simulink model "PhaseII_opalrt_NoProtection"  (Simulink 8.8)
settings: Solver=ode3  StartTime=0.0  StopTime=inf  FixedStep=Ts  RelTol=1e-5  EnableMultiTasking=on
PostLoadFcn:
  | %BESS ctrl
  | Kpf=0.005*3*12;
  | Kif=5*6;
  | 
  | Kpf1=0.005*3*12;
  | Kif1=5*6;
  | Kp_v=0.016*15*35;
  | Ki_v=12*25;
  | 
  | Kp_v1=0.016*15*35;
  | Ki_v1=12*25;
  | 
  | Vabc_B=12.47e3;
  | Vdc_ref=Vabc_B*2;
  | Kpwm=sqrt(2)*Vabc_B/Vdc_ref;
  | ZB=Vabc_B^2/1e6;
  | R=0.005*ZB;
  | Ibasefull=673/2*sqrt(2);
  | 
  | 
  | Ts_Control=1e-4;
  | ts=0.05;
  | delay=0.2;
  | offset=10e3;
  | t_plan=60;
  | t_monitor=.2;
  | t_mon=t_monitor;
  | scalingfactor=1;
  | x=0.5;
  | n=6;
  | %t_plan=1/15;
  | %t_monitor=10/900;
  | %t_mon=10/900;
  | 
  | %t_plan=1/5;
  | %t_monitor=10/300;
  | %t_mon=10/300;
  | %scalingfactor=1/300;
  | 
  | f0=60;
  | 
  | Pabc_B=1e6;
  | Iabc_B=Pabc_B*sqrt(2/3)/Vabc_B;  % pk value
  | Imax_1=2.5;
  | Ptrans_B=Pabc_B*200;
  | 
  | Vdc_ref=Vabc_B*2;
  | 
  | ZB=Vabc_B^2/Pabc_B;
  | L=0.1*ZB/2/pi/60;
  | R=0.1*ZB;
  | C=1/(4*pi^2*(2e3)^2*L);
  | 
  | LL=0.005*ZB/2/pi/60;
  | RR=0.005*ZB;
  | 
  | RC=0.02;
  | 
  | %%% Initial SOC %%%%
  | SOC_ini_BESS1=0.5;
  | ... (+223 lines)
InitFcn:
  | %BESS ctrl
  | Kpf=0.005*3*12;
  | Kif=5*6;
  | 
  | Kpf1=0.005*3*12;
  | Kif1=5*6;
  | Kp_v=0.016*15*35;
  | Ki_v=12*25;
  | 
  | Kp_v1=0.016*15*35;
  | Ki_v1=12*25;
  | 
  | Vabc_B=12.47e3;
  | Vdc_ref=Vabc_B*2;
  | Kpwm=sqrt(2)*Vabc_B/Vdc_ref;
  | ZB=Vabc_B^2/1e6;
  | R=0.005*ZB;
  | Ibasefull=673/2*sqrt(2);
  | 
  | 
  | Ts_Control=1e-4;
  | ts=0.05;
  | delay=0.2;
  | offset=10e3;
  | t_plan=60;
  | t_monitor=.2;
  | t_mon=t_monitor;
  | scalingfactor=1;
  | x=0.5;
  | n=6;
  | %t_plan=1/15;
  | %t_monitor=10/900;
  | %t_mon=10/900;
  | 
  | %t_plan=1/5;
  | %t_monitor=10/300;
  | %t_mon=10/300;
  | %scalingfactor=1/300;
  | 
  | f0=60;
  | 
  | Pabc_B=1e6;
  | Iabc_B=Pabc_B*sqrt(2/3)/Vabc_B;  % pk value
  | Imax_1=2.5;
  | Ptrans_B=Pabc_B*200;
  | 
  | Vdc_ref=Vabc_B*2;
  | 
  | ZB=Vabc_B^2/Pabc_B;
  | L=0.1*ZB/2/pi/60;
  | R=0.1*ZB;
  | C=1/(4*pi^2*(2e3)^2*L);
  | 
  | LL=0.005*ZB/2/pi/60;
  | RR=0.005*ZB;
  | 
  | RC=0.02;
  | 
  | %%% Initial SOC %%%%
  | SOC_ini_BESS1=0.5;
  | ... (+223 lines)
undefined symbols (not defined in the file): D1, Delta, DiscIntNeverNeededParam, Left, PG2ref, type, V
libraries: powerlib x220, powerlib_meascontrol x82, dspstat3 x54, dsparch4 x43, dspswit3 x24, simulink x19, simulink_extras x12, powerlib_extras x11, ssn_lib x7, artemis x6, rtlab x5, rtio_generic_dnp3 x5
(part 9 of 9)

== system PhaseII_opalrt_NoProtection/SM_System/Intellirupter/Intelliupter Measurement5/3Pto1P2 ==
  Vabc : Inport
  Demux9 : Demux  Outputs=3
  Gain : Gain  Gain=sqrt(2)
  Gain1 : Gain  Gain=sqrt(2)
  Gain2 : Gain  Gain=sqrt(2)
  Moving RMS : dspstat3/Moving RMS  Method=Exponential weighting  SpecifyWindowLength=off  WindowLength=4  ForgettingFactor=0.999  SimulateUsing=Code generation
  Moving RMS1 : dspstat3/Moving RMS  Method=Exponential weighting  SpecifyWindowLength=off  WindowLength=4  ForgettingFactor=0.999  SimulateUsing=Code generation
  Moving RMS2 : dspstat3/Moving RMS  Method=Exponential weighting  SpecifyWindowLength=off  WindowLength=4  ForgettingFactor=0.999  SimulateUsing=Code generation
  Va : Outport
  Vb : Outport  Port=2
  Vc : Outport  Port=3
  wires:
  Demux9/3 -> Moving RMS2/1
  Demux9/1 -> Moving RMS/1
  Demux9/2 -> Moving RMS1/1
  Vabc/1 -> Demux9/1
  Moving RMS/1 -> Gain/1
  Gain/1 -> Va/1
  Moving RMS1/1 -> Gain1/1
  Gain1/1 -> Vb/1
  Moving RMS2/1 -> Gain2/1
  Gain2/1 -> Vc/1

== system PhaseII_opalrt_NoProtection/SM_System/Intellirupter/Intelliupter Measurement5/Subsystem ==
  VaL : Inport
  VaR : Inport  Port=2
  VbL : Inport  Port=3
  VbR : Inport  Port=4
  VcL : Inport  Port=5
  VcR : Inport  Port=6
  Logical Operator : Logic  Inputs=3  AllPortsSameDT=off  OutDataTypeStr=boolean
  Relational Operator : RelationalOperator  Operator=<=  OutDataTypeStr=boolean  RndMeth=Simplest
  Relational Operator6 : RelationalOperator  Operator=<=  OutDataTypeStr=boolean  RndMeth=Simplest
  Relational Operator7 : RelationalOperator  Operator=<=  OutDataTypeStr=boolean  RndMeth=Simplest
  Subtract1 : Sum  Inputs=+-
  Subtract3 : Sum  Inputs=+-
  Subtract4 : Sum  Inputs=+-
  Vdiff : Outport
  wires:
  Subtract4/1 -> Relational Operator7/1
  Subtract3/1 -> Relational Operator6/1
  [V_mag_diff] -> Relational Operator7/2, Relational Operator6/2, Relational Operator/2
  Subtract1/1 -> Relational Operator/1
  VcR/1 -> Subtract4/2
  Relational Operator7/1 -> Logical Operator/3
  VcL/1 -> Subtract4/1
  VbL/1 -> Subtract3/1
  VbR/1 -> Subtract3/2
  Relational Operator/1 -> Logical Operator/1
  VaL/1 -> Subtract1/1
  VaR/1 -> Subtract1/2
  Relational Operator6/1 -> Logical Operator/2
  Logical Operator/1 -> Vdiff/1

== system PhaseII_opalrt_NoProtection/SM_System/Intellirupter/Intelliupter Measurement5/Subsystem1 ==
  VaL : Inport
  VbL : Inport  Port=2
  VcL : Inport  Port=3
  VaR : Inport  Port=4
  VbR : Inport  Port=5
  VcR : Inport  Port=6
  Logical Operator : Logic  Inputs=3  AllPortsSameDT=off  OutDataTypeStr=boolean
  Logical Operator1 : Logic  Inputs=3  AllPortsSameDT=off  OutDataTypeStr=boolean
  Relational Operator{3..4,6..9} (6 alike) : RelationalOperator  Operator=<=  OutDataTypeStr=boolean  RndMeth=Simplest
  VL : Outport
  VR : Outport  Port=2
  wires:
  [V_mag_limit] -> Relational Operator9/2, Relational Operator8/2, Relational Operator4/2, Relational Operator3/2, Relational Operator7/2, Relational Operator6/2
  VcL/1 -> Relational Operator4/1
  VaR/1 -> Relational Operator3/1
  Relational Operator4/1 -> Logical Operator/3
  Relational Operator6/1 -> Logical Operator/2
  VaL/1 -> Relational Operator7/1
  Relational Operator3/1 -> Logical Operator1/1
  VbL/1 -> Relational Operator6/1
  VcR/1 -> Relational Operator8/1
  Relational Operator9/1 -> Logical Operator1/2
  VbR/1 -> Relational Operator9/1
  Relational Operator7/1 -> Logical Operator/1
  Relational Operator8/1 -> Logical Operator1/3
  Logical Operator/1 -> VL/1
  Logical Operator1/1 -> VR/1

== system PhaseII_opalrt_NoProtection/SM_System/Intellirupter/Intelliupter Measurement6/3Pto1P1 ==
  Vabc : Inport
  Demux9 : Demux  Outputs=3
  Gain : Gain  Gain=sqrt(2)
  Gain1 : Gain  Gain=sqrt(2)
  Gain2 : Gain  Gain=sqrt(2)
  Moving RMS : dspstat3/Moving RMS  Method=Exponential weighting  SpecifyWindowLength=off  WindowLength=4  ForgettingFactor=0.999  SimulateUsing=Code generation
  Moving RMS1 : dspstat3/Moving RMS  Method=Exponential weighting  SpecifyWindowLength=off  WindowLength=4  ForgettingFactor=0.999  SimulateUsing=Code generation
  Moving RMS2 : dspstat3/Moving RMS  Method=Exponential weighting  SpecifyWindowLength=off  WindowLength=4  ForgettingFactor=0.999  SimulateUsing=Code generation
  Va : Outport
  Vb : Outport  Port=2
  Vc : Outport  Port=3
  wires:
  Demux9/3 -> Moving RMS2/1
  Demux9/1 -> Moving RMS/1
  Demux9/2 -> Moving RMS1/1
  Vabc/1 -> Demux9/1
  Moving RMS/1 -> Gain/1
  Gain/1 -> Va/1
  Moving RMS1/1 -> Gain1/1
  Gain1/1 -> Vb/1
  Moving RMS2/1 -> Gain2/1
  Gain2/1 -> Vc/1

== system PhaseII_opalrt_NoProtection/SM_System/Intellirupter/Intelliupter Measurement6/3Pto1P2 ==
  Vabc : Inport
  Demux9 : Demux  Outputs=3
  Gain : Gain  Gain=sqrt(2)
  Gain1 : Gain  Gain=sqrt(2)
  Gain2 : Gain  Gain=sqrt(2)
  Moving RMS : dspstat3/Moving RMS  Method=Exponential weighting  SpecifyWindowLength=off  WindowLength=4  ForgettingFactor=0.999  SimulateUsing=Code generation
  Moving RMS1 : dspstat3/Moving RMS  Method=Exponential weighting  SpecifyWindowLength=off  WindowLength=4  ForgettingFactor=0.999  SimulateUsing=Code generation
  Moving RMS2 : dspstat3/Moving RMS  Method=Exponential weighting  SpecifyWindowLength=off  WindowLength=4  ForgettingFactor=0.999  SimulateUsing=Code generation
  Va : Outport
  Vb : Outport  Port=2
  Vc : Outport  Port=3
  wires:
  Gain2/1 -> Vc/1
  Moving RMS2/1 -> Gain2/1
  Gain1/1 -> Vb/1
  Moving RMS1/1 -> Gain1/1
  Gain/1 -> Va/1
  Moving RMS/1 -> Gain/1
  Vabc/1 -> Demux9/1
  Demux9/2 -> Moving RMS1/1
  Demux9/1 -> Moving RMS/1
  Demux9/3 -> Moving RMS2/1

== system PhaseII_opalrt_NoProtection/SM_System/Intellirupter/Intelliupter Measurement6/Subsystem ==
  VaL : Inport
  VaR : Inport  Port=2
  VbL : Inport  Port=3
  VbR : Inport  Port=4
  VcL : Inport  Port=5
  VcR : Inport  Port=6
  Logical Operator : Logic  Inputs=3  AllPortsSameDT=off  OutDataTypeStr=boolean
  Relational Operator : RelationalOperator  Operator=<=  OutDataTypeStr=boolean  RndMeth=Simplest
  Relational Operator6 : RelationalOperator  Operator=<=  OutDataTypeStr=boolean  RndMeth=Simplest
  Relational Operator7 : RelationalOperator  Operator=<=  OutDataTypeStr=boolean  RndMeth=Simplest
  Subtract1 : Sum  Inputs=+-
  Subtract3 : Sum  Inputs=+-
  Subtract4 : Sum  Inputs=+-
  Vdiff : Outport
  wires:
  Logical Operator/1 -> Vdiff/1
  Relational Operator6/1 -> Logical Operator/2
  VaR/1 -> Subtract1/2
  VaL/1 -> Subtract1/1
  Relational Operator/1 -> Logical Operator/1
  VbR/1 -> Subtract3/2
  VbL/1 -> Subtract3/1
  VcL/1 -> Subtract4/1
  Relational Operator7/1 -> Logical Operator/3
  VcR/1 -> Subtract4/2
  Subtract1/1 -> Relational Operator/1
  [V_mag_diff] -> Relational Operator/2, Relational Operator6/2, Relational Operator7/2
  Subtract3/1 -> Relational Operator6/1
  Subtract4/1 -> Relational Operator7/1

== system PhaseII_opalrt_NoProtection/SM_System/Intellirupter/Intelliupter Measurement6/Subsystem1 ==
  VaL : Inport
  VbL : Inport  Port=2
  VcL : Inport  Port=3
  VaR : Inport  Port=4
  VbR : Inport  Port=5
  VcR : Inport  Port=6
  Logical Operator : Logic  Inputs=3  AllPortsSameDT=off  OutDataTypeStr=boolean
  Logical Operator1 : Logic  Inputs=3  AllPortsSameDT=off  OutDataTypeStr=boolean
  Relational Operator{3..4,6..9} (6 alike) : RelationalOperator  Operator=<=  OutDataTypeStr=boolean  RndMeth=Simplest
  VL : Outport
  VR : Outport  Port=2
  wires:
  Logical Operator1/1 -> VR/1
  Logical Operator/1 -> VL/1
  Relational Operator8/1 -> Logical Operator1/3
  Relational Operator7/1 -> Logical Operator/1
  VbR/1 -> Relational Operator9/1
  Relational Operator9/1 -> Logical Operator1/2
  VcR/1 -> Relational Operator8/1
  VbL/1 -> Relational Operator6/1
  Relational Operator3/1 -> Logical Operator1/1
  VaL/1 -> Relational Operator7/1
  Relational Operator6/1 -> Logical Operator/2
  Relational Operator4/1 -> Logical Operator/3
  VaR/1 -> Relational Operator3/1
  VcL/1 -> Relational Operator4/1
  [V_mag_limit] -> Relational Operator6/2, Relational Operator7/2, Relational Operator3/2, Relational Operator4/2, Relational Operator8/2, Relational Operator9/2

== system PhaseII_opalrt_NoProtection/SM_System/Intellirupter/Intelliupter Measurement7/3Pto1P1 ==
  Vabc : Inport
  Demux9 : Demux  Outputs=3
  Gain : Gain  Gain=sqrt(2)
  Gain1 : Gain  Gain=sqrt(2)
  Gain2 : Gain  Gain=sqrt(2)
  Moving RMS : dspstat3/Moving RMS  Method=Exponential weighting  SpecifyWindowLength=off  WindowLength=4  ForgettingFactor=0.999  SimulateUsing=Code generation
  Moving RMS1 : dspstat3/Moving RMS  Method=Exponential weighting  SpecifyWindowLength=off  WindowLength=4  ForgettingFactor=0.999  SimulateUsing=Code generation
  Moving RMS2 : dspstat3/Moving RMS  Method=Exponential weighting  SpecifyWindowLength=off  WindowLength=4  ForgettingFactor=0.999  SimulateUsing=Code generation
  Va : Outport
  Vb : Outport  Port=2
  Vc : Outport  Port=3
  wires:
  Gain2/1 -> Vc/1
  Moving RMS2/1 -> Gain2/1
  Gain1/1 -> Vb/1
  Moving RMS1/1 -> Gain1/1
  Gain/1 -> Va/1
  Moving RMS/1 -> Gain/1
  Vabc/1 -> Demux9/1
  Demux9/2 -> Moving RMS1/1
  Demux9/1 -> Moving RMS/1
  Demux9/3 -> Moving RMS2/1

== system PhaseII_opalrt_NoProtection/SM_System/Intellirupter/Intelliupter Measurement7/3Pto1P2 ==
  Vabc : Inport
  Demux9 : Demux  Outputs=3
  Gain : Gain  Gain=sqrt(2)
  Gain1 : Gain  Gain=sqrt(2)
  Gain2 : Gain  Gain=sqrt(2)
  Moving RMS : dspstat3/Moving RMS  Method=Exponential weighting  SpecifyWindowLength=off  WindowLength=4  ForgettingFactor=0.999  SimulateUsing=Code generation
  Moving RMS1 : dspstat3/Moving RMS  Method=Exponential weighting  SpecifyWindowLength=off  WindowLength=4  ForgettingFactor=0.999  SimulateUsing=Code generation
  Moving RMS2 : dspstat3/Moving RMS  Method=Exponential weighting  SpecifyWindowLength=off  WindowLength=4  ForgettingFactor=0.999  SimulateUsing=Code generation
  Va : Outport
  Vb : Outport  Port=2
  Vc : Outport  Port=3
  wires:
  Demux9/3 -> Moving RMS2/1
  Demux9/1 -> Moving RMS/1
  Demux9/2 -> Moving RMS1/1
  Vabc/1 -> Demux9/1
  Moving RMS/1 -> Gain/1
  Gain/1 -> Va/1
  Moving RMS1/1 -> Gain1/1
  Gain1/1 -> Vb/1
  Moving RMS2/1 -> Gain2/1
  Gain2/1 -> Vc/1

== system PhaseII_opalrt_NoProtection/SM_System/Intellirupter/Intelliupter Measurement7/Subsystem ==
  VaL : Inport
  VaR : Inport  Port=2
  VbL : Inport  Port=3
  VbR : Inport  Port=4
  VcL : Inport  Port=5
  VcR : Inport  Port=6
  Logical Operator : Logic  Inputs=3  AllPortsSameDT=off  OutDataTypeStr=boolean
  Relational Operator : RelationalOperator  Operator=<=  OutDataTypeStr=boolean  RndMeth=Simplest
  Relational Operator6 : RelationalOperator  Operator=<=  OutDataTypeStr=boolean  RndMeth=Simplest
  Relational Operator7 : RelationalOperator  Operator=<=  OutDataTypeStr=boolean  RndMeth=Simplest
  Subtract1 : Sum  Inputs=+-
  Subtract3 : Sum  Inputs=+-
  Subtract4 : Sum  Inputs=+-
  Vdiff : Outport
  wires:
  Subtract4/1 -> Relational Operator7/1
  Subtract3/1 -> Relational Operator6/1
  [V_mag_diff] -> Relational Operator7/2, Relational Operator6/2, Relational Operator/2
  Subtract1/1 -> Relational Operator/1
  VcR/1 -> Subtract4/2
  Relational Operator7/1 -> Logical Operator/3
  VcL/1 -> Subtract4/1
  VbL/1 -> Subtract3/1
  VbR/1 -> Subtract3/2
  Relational Operator/1 -> Logical Operator/1
  VaL/1 -> Subtract1/1
  VaR/1 -> Subtract1/2
  Relational Operator6/1 -> Logical Operator/2
  Logical Operator/1 -> Vdiff/1

== system PhaseII_opalrt_NoProtection/SM_System/Intellirupter/Intelliupter Measurement7/Subsystem1 ==
  VaL : Inport
  VbL : Inport  Port=2
  VcL : Inport  Port=3
  VaR : Inport  Port=4
  VbR : Inport  Port=5
  VcR : Inport  Port=6
  Logical Operator : Logic  Inputs=3  AllPortsSameDT=off  OutDataTypeStr=boolean
  Logical Operator1 : Logic  Inputs=3  AllPortsSameDT=off  OutDataTypeStr=boolean
  Relational Operator{3..4,6..9} (6 alike) : RelationalOperator  Operator=<=  OutDataTypeStr=boolean  RndMeth=Simplest
  VL : Outport
  VR : Outport  Port=2
  wires:
  [V_mag_limit] -> Relational Operator9/2, Relational Operator8/2, Relational Operator4/2, Relational Operator3/2, Relational Operator7/2, Relational Operator6/2
  VcL/1 -> Relational Operator4/1
  VaR/1 -> Relational Operator3/1
  Relational Operator4/1 -> Logical Operator/3
  Relational Operator6/1 -> Logical Operator/2
  VaL/1 -> Relational Operator7/1
  Relational Operator3/1 -> Logical Operator1/1
  VbL/1 -> Relational Operator6/1
  VcR/1 -> Relational Operator8/1
  Relational Operator9/1 -> Logical Operator1/2
  VbR/1 -> Relational Operator9/1
  Relational Operator7/1 -> Logical Operator/1
  Relational Operator8/1 -> Logical Operator1/3
  Logical Operator/1 -> VL/1
  Logical Operator1/1 -> VR/1

== system PhaseII_opalrt_NoProtection/SM_System/Intellirupter/Intelliupter Measurement8/3Pto1P1 ==
  Vabc : Inport
  Demux9 : Demux  Outputs=3
  Gain : Gain  Gain=sqrt(2)
  Gain1 : Gain  Gain=sqrt(2)
  Gain2 : Gain  Gain=sqrt(2)
  Moving RMS : dspstat3/Moving RMS  Method=Exponential weighting  SpecifyWindowLength=off  WindowLength=4  ForgettingFactor=0.999  SimulateUsing=Code generation
  Moving RMS1 : dspstat3/Moving RMS  Method=Exponential weighting  SpecifyWindowLength=off  WindowLength=4  ForgettingFactor=0.999  SimulateUsing=Code generation
  Moving RMS2 : dspstat3/Moving RMS  Method=Exponential weighting  SpecifyWindowLength=off  WindowLength=4  ForgettingFactor=0.999  SimulateUsing=Code generation
  Va : Outport
  Vb : Outport  Port=2
  Vc : Outport  Port=3
  wires:
  Demux9/3 -> Moving RMS2/1
  Demux9/1 -> Moving RMS/1
  Demux9/2 -> Moving RMS1/1
  Vabc/1 -> Demux9/1
  Moving RMS/1 -> Gain/1
  Gain/1 -> Va/1
  Moving RMS1/1 -> Gain1/1
  Gain1/1 -> Vb/1
  Moving RMS2/1 -> Gain2/1
  Gain2/1 -> Vc/1

== system PhaseII_opalrt_NoProtection/SM_System/Intellirupter/Intelliupter Measurement8/3Pto1P2 ==
  Vabc : Inport
  Demux9 : Demux  Outputs=3
  Gain : Gain  Gain=sqrt(2)
  Gain1 : Gain  Gain=sqrt(2)
  Gain2 : Gain  Gain=sqrt(2)
  Moving RMS : dspstat3/Moving RMS  Method=Exponential weighting  SpecifyWindowLength=off  WindowLength=4  ForgettingFactor=0.999  SimulateUsing=Code generation
  Moving RMS1 : dspstat3/Moving RMS  Method=Exponential weighting  SpecifyWindowLength=off  WindowLength=4  ForgettingFactor=0.999  SimulateUsing=Code generation
  Moving RMS2 : dspstat3/Moving RMS  Method=Exponential weighting  SpecifyWindowLength=off  WindowLength=4  ForgettingFactor=0.999  SimulateUsing=Code generation
  Va : Outport
  Vb : Outport  Port=2
  Vc : Outport  Port=3
  wires:
  Gain2/1 -> Vc/1
  Moving RMS2/1 -> Gain2/1
  Gain1/1 -> Vb/1
  Moving RMS1/1 -> Gain1/1
  Gain/1 -> Va/1
  Moving RMS/1 -> Gain/1
  Vabc/1 -> Demux9/1
  Demux9/2 -> Moving RMS1/1
  Demux9/1 -> Moving RMS/1
  Demux9/3 -> Moving RMS2/1

== system PhaseII_opalrt_NoProtection/SM_System/Intellirupter/Intelliupter Measurement8/Subsystem ==
  VaL : Inport
  VaR : Inport  Port=2
  VbL : Inport  Port=3
  VbR : Inport  Port=4
  VcL : Inport  Port=5
  VcR : Inport  Port=6
  Logical Operator : Logic  Inputs=3  AllPortsSameDT=off  OutDataTypeStr=boolean
  Relational Operator : RelationalOperator  Operator=<=  OutDataTypeStr=boolean  RndMeth=Simplest
  Relational Operator6 : RelationalOperator  Operator=<=  OutDataTypeStr=boolean  RndMeth=Simplest
  Relational Operator7 : RelationalOperator  Operator=<=  OutDataTypeStr=boolean  RndMeth=Simplest
  Subtract1 : Sum  Inputs=+-
  Subtract3 : Sum  Inputs=+-
  Subtract4 : Sum  Inputs=+-
  Vdiff : Outport
  wires:
  Logical Operator/1 -> Vdiff/1
  Relational Operator6/1 -> Logical Operator/2
  VaR/1 -> Subtract1/2
  VaL/1 -> Subtract1/1
  Relational Operator/1 -> Logical Operator/1
  VbR/1 -> Subtract3/2
  VbL/1 -> Subtract3/1
  VcL/1 -> Subtract4/1
  Relational Operator7/1 -> Logical Operator/3
  VcR/1 -> Subtract4/2
  Subtract1/1 -> Relational Operator/1
  [V_mag_diff] -> Relational Operator/2, Relational Operator6/2, Relational Operator7/2
  Subtract3/1 -> Relational Operator6/1
  Subtract4/1 -> Relational Operator7/1

== system PhaseII_opalrt_NoProtection/SM_System/Intellirupter/Intelliupter Measurement8/Subsystem1 ==
  VaL : Inport
  VbL : Inport  Port=2
  VcL : Inport  Port=3
  VaR : Inport  Port=4
  VbR : Inport  Port=5
  VcR : Inport  Port=6
  Logical Operator : Logic  Inputs=3  AllPortsSameDT=off  OutDataTypeStr=boolean
  Logical Operator1 : Logic  Inputs=3  AllPortsSameDT=off  OutDataTypeStr=boolean
  Relational Operator{3..4,6..9} (6 alike) : RelationalOperator  Operator=<=  OutDataTypeStr=boolean  RndMeth=Simplest
  VL : Outport
  VR : Outport  Port=2
  wires:
  Logical Operator1/1 -> VR/1
  Logical Operator/1 -> VL/1
  Relational Operator8/1 -> Logical Operator1/3
  Relational Operator7/1 -> Logical Operator/1
  VbR/1 -> Relational Operator9/1
  Relational Operator9/1 -> Logical Operator1/2
  VcR/1 -> Relational Operator8/1
  VbL/1 -> Relational Operator6/1
  Relational Operator3/1 -> Logical Operator1/1
  VaL/1 -> Relational Operator7/1
  Relational Operator6/1 -> Logical Operator/2
  Relational Operator4/1 -> Logical Operator/3
  VaR/1 -> Relational Operator3/1
  VcL/1 -> Relational Operator4/1
  [V_mag_limit] -> Relational Operator6/2, Relational Operator7/2, Relational Operator3/2, Relational Operator4/2, Relational Operator8/2, Relational Operator9/2

== system PhaseII_opalrt_NoProtection/SS_LocalControl/PV2/PLL /3-phase PLL1 ==
  note: Pierre Giroux, Gilbert Sybille
      | Power System Laboratory, IREQ
      | Hydro-Quebec
      | (August 2007)
  note: 3-phase PLL
  Vabc (pu) : Inport  PortDimensions=3
  2nd-Order Filter : powerlib_extras/Control  Blocks/2nd-Order Filter  FilterType=Lowpass  Fo=25  Zeta=0.707  Initialize=on  Vac_Init=[0 0 60]  Vdc_Init=Finit  PlotResponse=off  param1=[1 1000 0.5]
  Add : Sum
  Constant4 : Constant  Value=2*pi
  Discrete-Time Integrator : DiscreteIntegrator  gainval=1  InitialCondition=2*pi*Finit  InitialConditionSetting=State (most efficient)  SampleTime=-1  LimitOutput=on  UpperSaturationLimit=65*2*pi  LowerSaturationLimit=55*2*pi  ICPrevOutput=DiscIntNeverNeededParam  ICPrevScaledInput=DiscIntNeverNeededParam
  Gain10 : Gain  Gain=1/2/pi  SaturateOnIntegerOverflow=on  OutDataTypeStr=Inherit: Same as input  ParamDataTypeStr=Inherit: Same as input
  Integrator : Integrator  InitialCondition=Phase_Init*pi/180  LimitOutput=on
  Ki1 : Gain  Gain=Ki
  Kp1 : Gain  Gain=Kp
  Math Function : Math  Operator=mod  SaturateOnIntegerOverflow=on
  Mux2 : Mux  Inputs=2
  PID Controller : Subsystem  mask(PID Controller){Kp=Kp, Ki=Ki, Kd=Kd, Par_Limits=[10000 0], Init=2*pi*Finit}
      mask prompts: Kp "Proportional gain (Kp):"; Ki "Integral gain (Ki):"; Kd "Derivative gain (Kd):"; Par_Limits "Output limits: [ Upper   Lower ]"; Init "Output initial value:"
      mask help: This block implements a PID controller.
      mask init:
      | UpperLimit=Par_Limits(1);
      | LowerLimit=Par_Limits(2);
      mask Display: disp('PID');
  SW_Local1 : Scope  NumInputPorts=3
  Selector : Selector  InputPortWidth=3  IndexOptions=Index vector (dialog)  Indices=2  OutputSizes=1
  Trigonometric Function : Trigonometry
  Trigonometric Function2 : Trigonometry  Operator=cos
  abc_to_dq0 Transformation : powerlib_extras/Measurements/abc_to_dq0 Transformation
  Freq : Outport
  wt : Outport  Port=2
  Sin_Cos : Outport  Port=3
  Vdq0 : Outport  Port=4
  wires:
  Gain10/1 -> 2nd-Order Filter/1
  Mux2/1 -> abc_to_dq0 Transformation/2, Sin_Cos/1
  Trigonometric Function2/1 -> Mux2/2
  Trigonometric Function/1 -> Mux2/1
  Math Function/1 -> wt/1, Trigonometric Function2/1, Trigonometric Function/1
  Integrator/1 -> Math Function/1
  Constant4/1 -> Math Function/2
  abc_to_dq0 Transformation/1 -> Selector/1, Vdq0/1
  Vabc (pu)/1 -> abc_to_dq0 Transformation/1
  2nd-Order Filter/1 -> Freq/1
  Kp1/1 -> Add/1
  Ki1/1 -> Discrete-Time Integrator/1
  Discrete-Time Integrator/1 -> SW_Local1/3, Add/2
  Selector/1 -> SW_Local1/1, Kp1/1, Ki1/1  "Vq"
  Add/1 -> Gain10/1, SW_Local1/2, Integrator/1

== system PhaseII_opalrt_NoProtection/SS_LocalControl/PV2/PLL /VLtoVphase6 ==
  VLabc : Inport
  Mux : Mux  Inputs=[3]
  Mux1 : Mux  Inputs=3
  dq2alpha : Fcn  Expr=(2*u[1]+u[2])/3
  dq2beta : Fcn  Expr=(2*u[2]+u[3])/3
  dq2beta1 : Fcn  Expr=(2*u[3]+u[1])/3
  Vph_abc : Outport
  wires:
  dq2beta1/1 -> Mux1/3
  VLabc/1 -> Mux/1
  Mux/1 -> dq2beta1/1, dq2beta/1, dq2alpha/1
  dq2alpha/1 -> Mux1/1
  dq2beta/1 -> Mux1/2
  Mux1/1 -> Vph_abc/1

== system PhaseII_opalrt_NoProtection/SS_LocalControl/PV2/PLL /3-phase PLL1/PID Controller ==
  Error : Inport
  Derivative : Derivative
  Integrator : Integrator  InitialCondition=Init  LimitOutput=on  UpperSaturationLimit=UpperLimit  LowerSaturationLimit=LowerLimit
  Kp1 : Gain  Gain=Kd  SaturateOnIntegerOverflow=on  OutDataTypeStr=Inherit: Same as input  ParamDataTypeStr=Inherit: Same as input
  Kp4 : Gain  Gain=Kp  SaturateOnIntegerOverflow=on  OutDataTypeStr=Inherit: Same as input  ParamDataTypeStr=Inherit: Same as input
  Kp5 : Gain  Gain=Ki  SaturateOnIntegerOverflow=on  OutDataTypeStr=Inherit: Same as input  ParamDataTypeStr=Inherit: Same as input
  Saturation2 : Saturate  UpperLimit=UpperLimit  LowerLimit=LowerLimit
  Sum6 : Sum  Inputs=+++  SaturateOnIntegerOverflow=on  InputSameDT=on  OutDataTypeStr=Inherit: Same as first input
  Out : Outport  InitialOutput=0
  wires:
  Saturation2/1 -> Out/1
  Integrator/1 -> Sum6/2
  Kp4/1 -> Sum6/1
  Kp5/1 -> Integrator/1
  Sum6/1 -> Saturation2/1
  Error/1 -> Kp5/1, Kp4/1, Kp1/1
  Kp1/1 -> Derivative/1
  Derivative/1 -> Sum6/3

== matlab function SS_LocalControl/BESS1/PI_Vd3/Embedded MATLAB Function1 ==
  data: dout output double; din input double; enable input double
function dout = fcn(din,enable)
if enable==1
    dout=din;
else
    dout=double(0);
end

== matlab function SS_LocalControl/BESS1/PI_Vd1/Embedded MATLAB Function1 ==
  data: dout output double; din input double; enable input double
function dout = fcn(din,enable)
if enable==1
    dout=din;
else
    dout=double(0);
end

== matlab function SS_LocalControl/BESS1/PI_Vd2/Embedded MATLAB Function1 ==
  data: dout output double; din input double; enable input double
function dout = fcn(din,enable)
if enable==1
    dout=din;
else
    dout=double(0);
end

== matlab function SS_LocalControl/PV2/PI_daxis1/Embedded MATLAB Function1 ==
  data: dout output double; din input double; enable input double
function dout = fcn(din,enable)
if enable==1
    dout=din;
else
    dout=double(0);
end

== matlab function SS_LocalControl/PV2/PI_daxis2/Embedded MATLAB Function1 ==
  data: dout output double; din input double; enable input double
function dout = fcn(din,enable)
if enable==1
    dout=din;
else
    dout=double(0);
end

== matlab function SS_LocalControl/BESS1/PI_Vd5/Embedded MATLAB Function1 ==
  data: dout output double; din input double; enable input double
function dout = fcn(din,enable)
if enable==1
    dout=din;
else
    dout=double(0);
end

== matlab function SS_LocalControl/BESS1/PI_Vd6/Embedded MATLAB Function1 ==
  data: dout output double; din input double; enable input double
function dout = fcn(din,enable)
if enable==1
    dout=din;
else
    dout=double(0);
end

== matlab function SS_LocalControl/BESS1/PI_Vd8/Embedded MATLAB Function1 ==
  data: dout output double; din input double; enable input double
function dout = fcn(din,enable)
if enable==1
    dout=din;
else
    dout=double(0);
end

== matlab function SM_System/Generator2/PI_Vd10/Embedded MATLAB Function1 ==
  data: dout output double; din input double; enable input double
function dout = fcn(din,enable)
if enable==1
    dout=din;
else
    dout=double(0);
end

== matlab function SS_LocalControl/BESS1/PI_Vd10/Embedded MATLAB Function1 ==
  data: dout output double; din input double; enable input double
function dout = fcn(din,enable)
if enable==1
    dout=din;
else
    dout=double(0);
end

== matlab function SS_LocalControl/BESS2/PI_Vd10/Embedded MATLAB Function1 ==
  data: dout output double; din input double; enable input double
function dout = fcn(din,enable)
if enable==1
    dout=din;
else
    dout=double(0);
end

== matlab function SS_LocalControl/BESS2/PI_Vd2/Embedded MATLAB Function1 ==
  data: dout output double; din input double; enable input double
function dout = fcn(din,enable)
if enable==1
    dout=din;
else
    dout=double(0);
end

== matlab function SS_LocalControl/BESS1/PI_Vd7/Embedded MATLAB Function1 ==
  data: dout output double; din input double; enable input double
function dout = fcn(din,enable)
if enable==1
    dout=din;
else
    dout=double(0);
end

== matlab function SS_LocalControl/BESS1/PI_Vd9/Embedded MATLAB Function1 ==
  data: dout output double; din input double; enable input double
function dout = fcn(din,enable)
if enable==1
    dout=din;
else
    dout=double(0);
end

== matlab function SS_LocalControl/BESS2/PI_Vd1/Embedded MATLAB Function1 ==
  data: dout output double; din input double; enable input double
function dout = fcn(din,enable)
if enable==1
    dout=din;
else
    dout=double(0);
end

== matlab function SS_LocalControl/BESS1/PI_Vd11/Embedded MATLAB Function1 ==
  data: dout output double; din input double; enable input double
function dout = fcn(din,enable)
if enable==1
    dout=din;
else
    dout=double(0);
end

== matlab function SS_LocalControl/BESS2/PI_Vd3/Embedded MATLAB Function1 ==
  data: dout output double; din input double; enable input double
function dout = fcn(din,enable)
if enable==1
    dout=din;
else
    dout=double(0);
end

== matlab function SM_System/Generator2/PI_Vd1/Embedded MATLAB Function1 ==
  data: dout output double; din input double; enable input double
function dout = fcn(din,enable)
if enable==1
    dout=din;
else
    dout=double(0);
end

== matlab function SM_System/Generator2/Embedded MATLAB Function1 ==
  data: dout output double; din input double; fbkin input double; enable input double
function dout  = fcn(din,fbkin, enable)
if enable==1
    dout=fbkin*0.999;
else
    dout=din;
end

== matlab function SS_LocalControl/BESS2/PI_Vd4/Embedded MATLAB Function1 ==
  data: dout output double; din input double; enable input double
function dout = fcn(din,enable)
if enable==1
    dout=din;
else
    dout=double(0);
end

== matlab function SS_LocalControl/BESS2/PI_Vd5/Embedded MATLAB Function1 ==
  data: dout output double; din input double; enable input double
function dout = fcn(din,enable)
if enable==1
    dout=din;
else
    dout=double(0);
end

== matlab function SS_LocalControl/BESS2/PI_Vd6/Embedded MATLAB Function1 ==
  data: dout output double; din input double; enable input double
function dout = fcn(din,enable)
if enable==1
    dout=din;
else
    dout=double(0);
end

== matlab function SS_LocalControl/BESS2/PI_Vd7/Embedded MATLAB Function1 ==
  data: dout output double; din input double; enable input double
function dout = fcn(din,enable)
if enable==1
    dout=din;
else
    dout=double(0);
end

== matlab function SS_LocalControl/BESS2/PI_Vd8/Embedded MATLAB Function1 ==
  data: dout output double; din input double; enable input double
function dout = fcn(din,enable)
if enable==1
    dout=din;
else
    dout=double(0);
end

== matlab function SS_LocalControl/BESS2/PI_Vd9/Embedded MATLAB Function1 ==
  data: dout output double; din input double; enable input double
function dout = fcn(din,enable)
if enable==1
    dout=din;
else
    dout=double(0);
end
